simulink model "logicchargingtesting"  (R2023b)
settings: Solver=VariableStepAuto  StartTime=0.0  StopTime=100  RelTol=1e-3
settings Model: Creator=lricc  LastModifiedBy=lricc

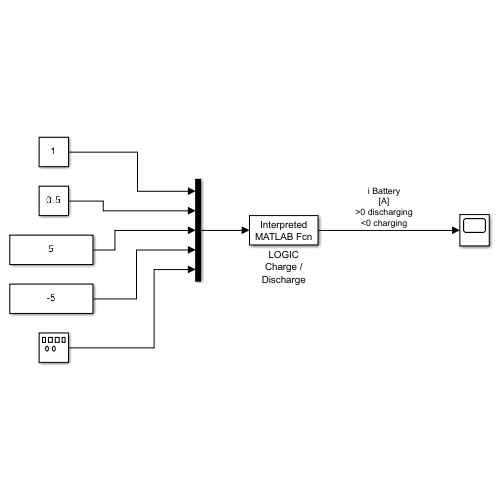
[thumbnail: Simulink's stored preview of the top-level diagram]
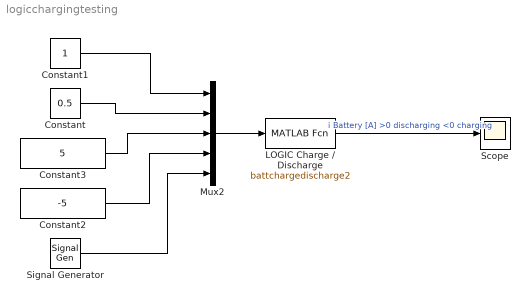
== system logicchargingtesting ==
  Constant : Constant  Value=0.5
  Constant1 : Constant
  Constant2 : Constant  Value=-5
  Constant3 : Constant  Value=5
  LOGIC Charge / Discharge : MATLABFcn  MATLABFcn=battchargedischarge2
  Mux2 : Mux  Inputs=5
  Scope : Scope
  Signal Generator : SignalGenerator  WaveForm=sawtooth  Amplitude=5  Frequency=0.05  Units=rad/sec
  wires:
  Constant1/1 -> Mux2/1
  Constant3/1 -> Mux2/3
  Constant2/1 -> Mux2/4
  Signal Generator/1 -> Mux2/5
  Mux2/1 -> LOGIC Charge / Discharge/1
  Constant/1 -> Mux2/2
  LOGIC Charge / Discharge/1 -> Scope/1  "i Battery [A] >0 discharging <0 charging"
